simulink model "FinalProject"  (R2023a)
settings: Solver=ode1be  StartTime=0.0  StopTime=10  RelTol=1e-3
settings Model: Creator=romav  LastModifiedBy=mrrom

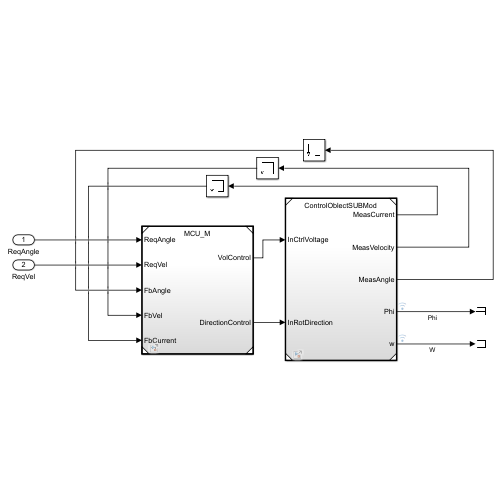
[thumbnail: Simulink's stored preview of the top-level diagram]
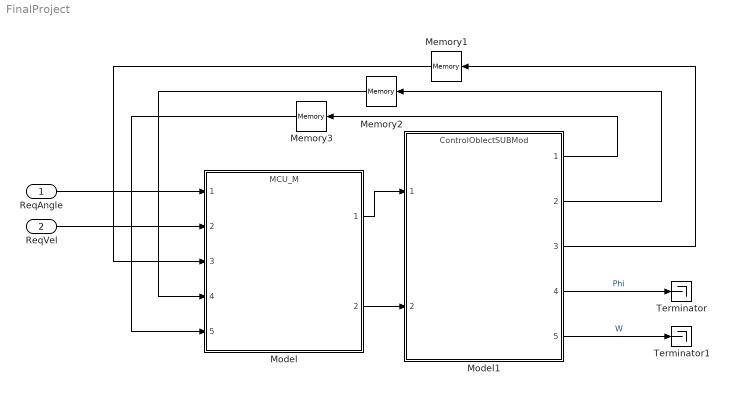
== system FinalProject ==
  ReqAngle : Inport
  ReqVel : Inport  Port=2
  Memory1 : Memory
  Memory2 : Memory
  Memory3 : Memory
  Model : ModelReference  ModelNameDialog=MCU_M.slx  SimulationMode=Normal  ModelReferenceVersion=1.7
  Model1 : ModelReference  ModelNameDialog=ControlOblectSUBMod.slx  SimulationMode=Normal  ModelReferenceVersion=1.13
  Terminator : Terminator
  Terminator1 : Terminator
  wires:
  Model/1 -> Model1/1
  Model/2 -> Model1/2
  Model1/1 -> Memory3/1
  Model1/2 -> Memory2/1
  Model1/3 -> Memory1/1
  Memory1/1 -> Model/3
  Memory2/1 -> Model/4
  Memory3/1 -> Model/5
  ReqAngle/1 -> Model/1
  Model1/4 -> Terminator/1  "Phi"
  Model1/5 -> Terminator1/1  "W"
  ReqVel/1 -> Model/2
